simulink model "Rover"  (R2023b)
settings: Solver=FixedStepDiscrete  StartTime=0.0  StopTime=1000  RelTol=1e-3  EnableMultiTasking=on
model workspace (MAT data in the model file):
  state_1 = 0
(part 1 of 2)
settings Model: ExtModeTrigDuration=10  Creator=teodo  LastModifiedBy=anton
settings OptimizationCC: UseDivisionForNetSlopeComputation=on  GainParamInheritBuiltInType=on  UseFloatMulNetSlope=on  OptimizeBlockIOStorage=off  BufferReuse=off  ReuseModelBlockBuffer=off  GlobalBufferReuse=off  ExpressionFolding=off  EnableMemcpy=off  PassReuseOutputArgsAs=Individual arguments  LocalBlockOutputs=off  ZeroExternalMemoryAtStartup=off  ZeroInternalMemoryAtStartup=off  NoFixptDivByZeroProtection=on  EfficientFloat2IntCast=on  LifeSpan=1  MaxStackSize=64  OptimizeDataStoreBuffers=off  BusAssignmentInplaceUpdate=off  OptimizationLevel=level0  OptimizationCustomize=off  EfficientTunableParamExpr=on
settings DebuggingCC: ParameterPrecisionLossMsg=none  ParameterTunabilityLossMsg=error
settings HardwareCC: ProdBitPerPointer=32  ProdBitPerSizeT=32  ProdBitPerPtrDiffT=32  ProdLargestAtomicInteger=Long  ProdLargestAtomicFloat=Double  ProdWordSize=32  ProdLongLongMode=on  ProdHWDeviceType=ARM Compatible->ARM Cortex
settings SFSimCC: MATLABDynamicMemAlloc=off
settings RTWCC: Description=Embedded Coder  SystemTargetFile=ert.tlc  HardwareBoard=STM32 Nucleo F401RE  TemplateMakefile=ert_default_tmf  Toolchain=GNU Tools for ARM Embedded Processors  CodeExecutionProfiling=on  CodeProfilingSaveOptions=AllData  CodeProfilingInstrumentation=detailed
settings CodeAppCC: ForceParamTrailComments=on  IgnoreCustomStorageClasses=off  OperatorAnnotations=on  SimulinkDataObjDesc=on  SFDataObjDesc=on  CustomSymbolStrGlobalVar=rt$N$M  CustomSymbolStrType=$N$M  CustomSymbolStrFcn=$N$M$F  CustomSymbolStrMacro=$N$M  InsertBlockDesc=on
settings ERTTargetCC: IncludeMdlTerminateFcn=off  CombineSignalStateStructs=on  SupportAbsoluteTime=off  CodeInterfacePackaging=Reusable function  SupportNonFinite=off  SupportComplex=off  SupportNonInlinedSFcns=on  ExtModeTransport=3  ExtModeStaticAlloc=on  ExtModeStaticAllocSize=2000  ExtModeMexFile=ext_xcp  ExtModeIntrfLevel=Level2 - Open  ERTFilePackagingFormat=CompactWithDataFile

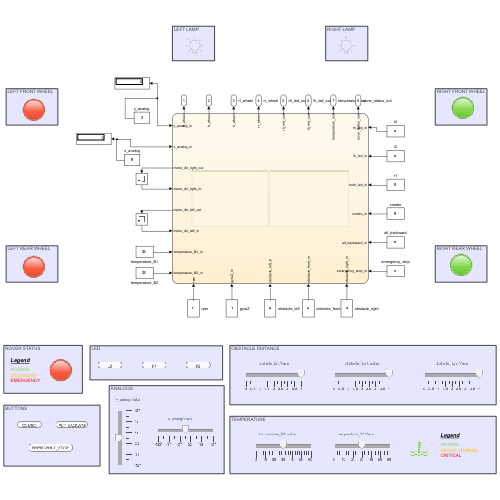
[thumbnail: Simulink's stored preview of the top-level diagram]
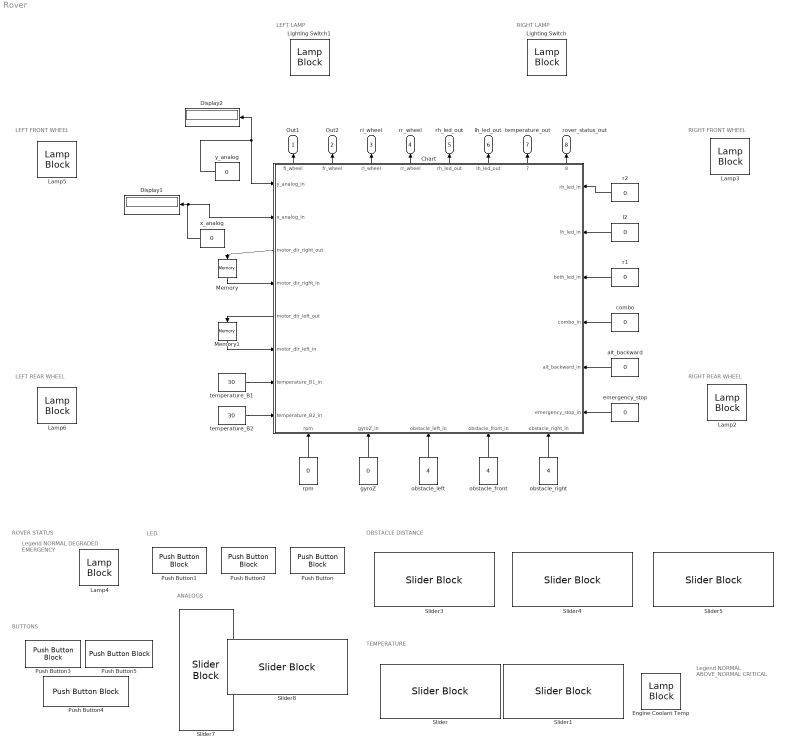
== system Rover ==
  note: LEFT LAMP
  note: BUTTONS
  note: Legend
      |
      | NORMAL
      | DEGRADED
      | EMERGENCY
  note: ROVER STATUS
  note: OBSTACLE DISTANCE
  note: TEMPERATURE
  note: ANALOGS
  note: LED
  note: Legend
      |
      | NORMAL
      | ABOVE_NORMAL
      | CRITICAL
  note: RIGHT FRONT WHEEL
  note: RIGHT REAR WHEEL
  note: RIGHT LAMP
  note: LEFT FRONT WHEEL
  note: LEFT REAR WHEEL
  Chart : Stateflow chart  TreatAsAtomicUnit=on
      settings: PortSchema="{\"entries\":[{\"content\":{\"sides\":[{\"content\":{\"connectorIds\":[\"In8\",\"In9\",\"Out9\",\"In1\",\"Out10\",\"In2\",\"In3\",\"In4\"]},\"type\":\"ConnectorPlacement.EquallySpacedRectSide\",\"uuid\":\"7cce3b45-ffbe-4cab-b07c-1dbc7baad8c5\"},{\"content\":{\"connectorIds\":[\"In10\",\"In11\",\"In12\",\"In13\",\"In14\",\"In15\"],\"side\":\"RIGHT\"},\"type\":\"ConnectorPlacement.EquallySpacedRectSide\",\"uuid\":\"3e6480be-640f-4a32-82b3-6b3437d92763\"},{\"content\":{\"connectorIds\":[\"Out1\",\"Out2\",\"Out3\",\"Out4\",\"Out5\",\"Out6\",\"Out7\",\"Out8\"],\"side\":\"TOP\"},\"type\":\"ConnectorPlacement.EquallySpacedRectSide\",\"uuid\":\"fd9d4029-269d-4faa-a5ce-8ba36361a7f1\"},{\"content\":{\"connectorIds\":[\"In17\",\"In16\",\"In5\",\"In6\",\"In7\"],\"side\":\"BOTTOM\"},\"type\":\"ConnectorPlacement.EquallySpacedRectSide\",\"uuid\":\"6525cc66-ebfe-4a16-99cf-a0e40f8056c2\"}]},\"type\":\"ConnectorPlacement.EquallySpacedConnector\",\"uuid\":\"44bb7497-2c81-49aa-af62-cacbc00a1727\"}],\"packageUris\":[\"http://schema.mathworks.com/mf0/Connector/R2020b\"],\"version\":\"1.0\"}"
  Display1 : Display
  Display2 : Display
  Engine Coolant Temp : LampBlock  LabelPosition=Hide  Icon=EngineCoolantTemp
  Lamp{2..6} (5 alike) : LampBlock  LabelPosition=Hide
  Lighting Switch : LampBlock  LabelPosition=Hide  Icon=LightingSwitch
  Lighting Switch1 : LampBlock  LabelPosition=Hide  Icon=LightingSwitch
  Memory : Memory
  Memory1 : Memory
  Push Button : PushButtonBlock  ButtonText=R2  OffValue=0.000000
  Push Button1 : PushButtonBlock  ButtonText=L2  OffValue=0.000000
  Push Button2 : PushButtonBlock  ButtonText=R1  OffValue=0.000000
  Push Button3 : PushButtonBlock  ButtonText=COMBO  ButtonType=Latch  OffValue=0.000000
  Push Button4 : PushButtonBlock  ButtonText=EMERGENCY_STOP  OffValue=0.000000
  Push Button5 : PushButtonBlock  ButtonText=ALT_BACKWARD  OffValue=0.000000
  Slider : SliderBlock  ScaleMax=60
  Slider1 : SliderBlock  ScaleMax=60
  Slider3 : SliderBlock  ScaleMax=4
  Slider4 : SliderBlock  ScaleMax=4
  Slider5 : SliderBlock  ScaleMax=4
  Slider7 : SliderBlock  ScaleMin=-127  ScaleMax=127
  Slider8 : SliderBlock  ScaleMin=-127  ScaleMax=127
  alt_backward : Constant  Value=0  OutDataTypeStr=uint8
  combo : Constant  Value=0  OutDataTypeStr=uint8
  emergency_stop : Constant  Value=0  OutDataTypeStr=uint8
  gyroZ : Constant  Value=0
  l2 : Constant  Value=0  OutDataTypeStr=uint8
  obstacle_front : Constant  Value=4
  obstacle_left : Constant  Value=4
  obstacle_right : Constant  Value=4
  r1 : Constant  Value=0  OutDataTypeStr=uint8
  r2 : Constant  Value=0  OutDataTypeStr=uint8
  rpm : Constant  Value=0
  temperature_B1 : Constant  Value=30
  temperature_B2 : Constant  Value=30
  x_analog : Constant  Value=0  OutDataTypeStr=int8
  y_analog : Constant  Value=0  OutDataTypeStr=int8
  Out1 : Outport
  Out2 : Outport  Port=2
  rl_wheel : Outport  Port=3
  rr_wheel : Outport  Port=4
  rh_led_out : Outport  Port=5
  lh_led_out : Outport  Port=6
  temperature_out : Outport  Port=7
  rover_status_out : Outport  Port=8
  wires:
  temperature_B1/1 -> Chart/3(temperature_B1_in)
  temperature_B2/1 -> Chart/4(temperature_B2_in)
  obstacle_left/1 -> Chart/5(obstacle_left_in)
  obstacle_front/1 -> Chart/6(obstacle_front_in)
  obstacle_right/1 -> Chart/7(obstacle_right_in)
  y_analog/1 -> Display2/1, Chart/8(y_analog_in)
  Chart/1(fl_wheel) -> Out1/1
  Chart/2(fr_wheel) -> Out2/1
  Chart/3(rl_wheel) -> rl_wheel/1
  Chart/4(rr_wheel) -> rr_wheel/1
  Chart/5(rh_led_out) -> rh_led_out/1
  Chart/6(lh_led_out) -> lh_led_out/1
  r2/1 -> Chart/10(rh_led_in)
  l2/1 -> Chart/11(lh_led_in)
  r1/1 -> Chart/12(both_led_in)
  x_analog/1 -> Chart/9(x_analog_in), Display1/1
  Chart/7(temperature_out) -> temperature_out/1
  Chart/8(rover_status_out) -> rover_status_out/1
  combo/1 -> Chart/13(combo_in)
  alt_backward/1 -> Chart/14(alt_backward_in)
  emergency_stop/1 -> Chart/15(emergency_stop_in)
  gyroZ/1 -> Chart/16(gyroZ_in)
  Chart/9(motor_dir_right_out) -> Memory/1
  Chart/10(motor_dir_left_out) -> Memory1/1
  Memory/1 -> Chart/1(motor_dir_right_in)
  Memory1/1 -> Chart/2(motor_dir_left_in)
  rpm/1 -> Chart/17(rpm)
